simulink model "SRFF_MS"  (R2025a)
settings: Solver=VariableStepAuto  StartTime=0.0  StopTime=Inf  RelTol=1e-3
settings Model: Creator=Soochan Kim  LastModifiedBy=Soochan Kim

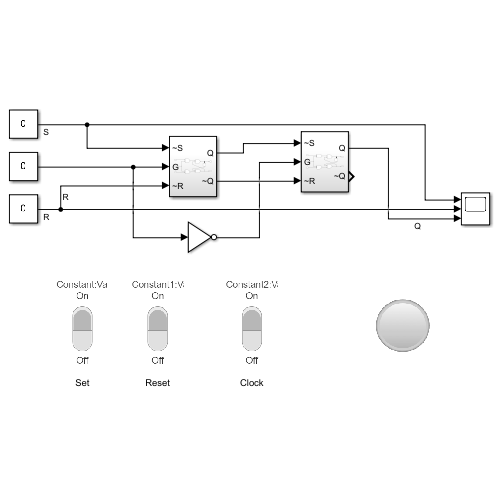
[thumbnail: Simulink's stored preview of the top-level diagram]
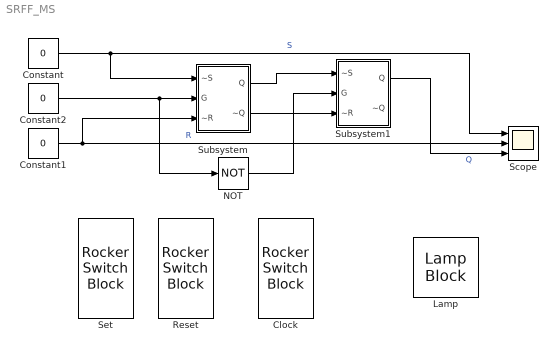
== system SRFF_MS ==
  Clock : RockerSwitchBlock
  Constant : Constant  Value=0
  Constant1 : Constant  Value=0
  Constant2 : Constant  Value=0
  Lamp : LampBlock  LabelPosition=Hide  DefaultColor=[192.0, 192.0, 192.0]
  NOT : Logic  Operator=NOT  IconShape=distinctive  AllPortsSameDT=off  OutDataTypeStr=boolean
  Reset : RockerSwitchBlock
  Scope : Scope  NumInputPorts=3
      settings: ActiveDisplayYMinimum=-1  ActiveDisplayYMaximum=1.125
  Set : RockerSwitchBlock
  Subsystem : Subsystem
  Subsystem1 : Subsystem
  wires:
  Constant/1 -> Subsystem/1(~S), Scope/1  "S"
  Constant2/1 -> NOT/1, Subsystem/2(G)
  Subsystem/1(Q) -> Subsystem1/1(~S)
  Subsystem/2(~Q) -> Subsystem1/3(~R)
  NOT/1 -> Subsystem1/2(G)
  Subsystem1/1(Q) -> Scope/3  "Q"
  Constant1/1 -> Subsystem/3(~R), Scope/2  "R"

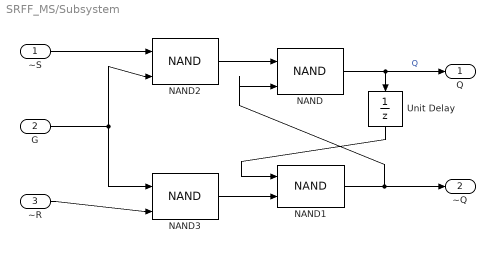
== system SRFF_MS/Subsystem ==
  ~S : Inport
  G : Inport  Port=2
  ~R : Inport  Port=3
  NAND{,1..3} (4 alike) : Logic  Operator=NAND  IconShape=distinctive  AllPortsSameDT=off  OutDataTypeStr=boolean
  Unit Delay : UnitDelay  SampleTime=-1  HasFrameUpgradeWarning=on
  Q : Outport
  ~Q : Outport  Port=2
  wires:
  Unit Delay/1 -> NAND1/1
  NAND1/1 -> ~Q/1, NAND/2
  G/1 -> NAND2/2, NAND3/1
  ~R/1 -> NAND3/2
  NAND2/1 -> NAND/1
  NAND/1 -> Q/1, Unit Delay/1  "Q"
  NAND3/1 -> NAND1/2
  ~S/1 -> NAND2/1

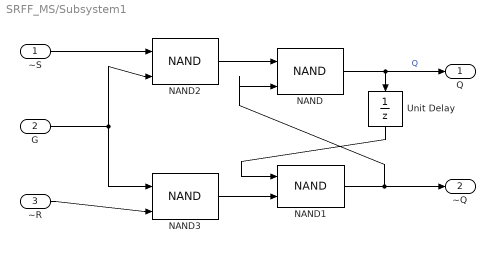
== system SRFF_MS/Subsystem1 ==
  ~S : Inport
  G : Inport  Port=2
  ~R : Inport  Port=3
  NAND{,1..3} (4 alike) : Logic  Operator=NAND  IconShape=distinctive  AllPortsSameDT=off  OutDataTypeStr=boolean
  Unit Delay : UnitDelay  SampleTime=-1  HasFrameUpgradeWarning=on
  Q : Outport
  ~Q : Outport  Port=2
  wires:
  Unit Delay/1 -> NAND1/1
  NAND1/1 -> ~Q/1, NAND/2
  G/1 -> NAND2/2, NAND3/1
  ~R/1 -> NAND3/2
  NAND2/1 -> NAND/1
  NAND/1 -> Q/1, Unit Delay/1  "Q"
  NAND3/1 -> NAND1/2
  ~S/1 -> NAND2/1
